simulink model "work_SensorModel"  (R2026a)
settings: Solver=FixedStepAuto  StartTime=0  StopTime=1000  FixedStep=simStepSize
settings Model: Creator=The MathWorks, Inc.  LastModifiedBy=akshran
settings DataIOCC: MaxDataPoints=100  SaveFormat=StructureWithTime  DatasetSignalFormat=timetable
settings DebuggingCC: SubsystemReferenceDiagnosticForUnitTest=warning

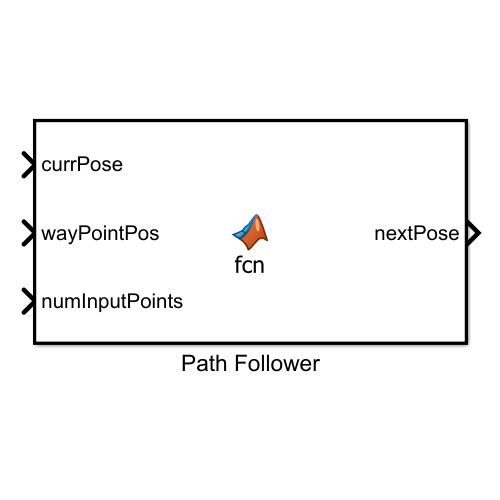
[thumbnail: Simulink's stored preview of the top-level diagram]
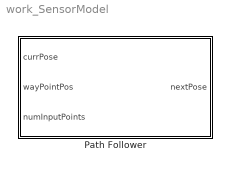
== system work_SensorModel ==
  Path Follower : MATLAB Function  TreatAsAtomicUnit=on

== matlab function work_SensorModel/Path Follower ==
  data: currPose input; wayPointPos input; numInputPoints input; nextPose output Bus: BusActorRuntime; simStepSize parameter
function nextPose = fcn(currPose, wayPointPos, numInputPoints, simStepSize)

% Set constant ego vehicle speed
egoSpeed  = 18;

% Declare persistent variables for simulation and retain only non zero
% elements in the array of waypoints 
persistent wayPointIdx wayPointPosInterp headingAnglesInterp numWayPoints
wayPointPos = wayPointPos(1:numInputPoints,:);

% Extract poses for the entire path before simulation begins
if isempty(wayPointIdx)
    
    wayPointIdx = 2;

    % Pre-allocate arrays
    wayPointPosInterp = [];
    headingAnglesInterp = [];

    % Get heading angle
    startHeadingAngle = atan2d(-currPose.Pose(1,2),currPose.Pose(1,1));
  
     % Calculate distance from the each waypoint to the next waypoint
    delXY = diff(wayPointPos(:,[1 2]));
    absDistToNextPoints = sqrt(delXY(:,1).^2 + delXY(:,2).^2);

    % Calculate time of arrival at the next wayPoint based on the
    % set constant speed. Alternatively, you can set the timing profile
    % in RoadRunner for waypoints and use those here 
    trueTimes = [0;cumsum(absDistToNextPoints/egoSpeed)];

    % Calculate the heading angle to proceed towards each waypoint
    headingAngles = [startHeadingAngle;atan2d(delXY(:,2),delXY(:,1))-90];

    % Calculate time of arrival at all the wayPoints based on the
    % simulation step size and use it for final interpolation.
    globalTimeVec = 0:simStepSize:trueTimes(end);

    % Interpolate X and Y positions between all waypoints
    % along the entire time vector and store them
    interpPosPointsX = interp1(trueTimes,wayPointPos(:,1),globalTimeVec)';
    interpPosPointsY = interp1(trueTimes,wayPointPos(:,2),globalTimeVec)';
    wayPointPosInterp = [interpPosPointsX interpPosPointsY];

    % Interpolate heading angles between the all waypoints
    % along the entire time vector and store them
    headingAnglesInterp = interp1(trueTimes,headingAngles,globalTimeVec');

    % Get the new total number of waypoints after interpolation
    numWayPoints = length(wayPointPosInterp);
end

% At each time step of the simulation, send the next waypoint position from the
% interpolated waypoint array until ego vehicle arrives at the last waypoint
nextPose = currPose;
nextPose.Pose(1,4) = wayPointPosInterp(wayPointIdx,1);
nextPose.Pose(2,4) = wayPointPosInterp(wayPointIdx,2);

% Convert the heading angle (yaw) to a rotation matrix
nextPose.Pose(1:3,1:3) = [cosd(headingAnglesInterp(wayPointIdx)) -sind(headingAnglesInterp(wayPointIdx)) 0;...
                          sind(headingAnglesInterp(wayPointIdx)) cosd(headingAnglesInterp(wayPointIdx)) 0;...
                          0 0 1];

if(wayPointIdx<numWayPoints)
    wayPointIdx = wayPointIdx + 1;
end

end
